simulink model "simRelativeNavSurfelGridMap"  (R2020b)
settings: Solver=FixedStepAuto  StartTime=0.0  StopTime=tEnd  FixedStep=dtSim  RelTol=1e-3
values from neighbouring files (symbols this model uses):
  flagUseTrueRelStates = 0    [testEnvironmentV2.m]    (also in testEnvironments.m = 1; testEnvironmentsV2.m; testEnvironmentsV3.m)
  fLArrayDim = size(fL1MeasArrayDir,1)    [SurfelGridMap.m]    (also in testEnvironmentV2.m = 256; testEnvironments.m = 256; testEnvironmentsV2.m = 256; testEnvironmentsV3.m = 256)
undefined symbols (not defined in the file or in its folder): angRate_IT_T, covMeasNoise, covProcessNoise, dtSim, fL1Pose_B, flagGravityAlignedNode, initCovState, initX, paramSGM, posi_TL_T, quat_TL, tEnd
libraries: IMUUnit x1, flashLiDARUnit x1
(part 2 of 2)

== matlab function simRelativeNavSurfelGridMap/RNerrorStateKalmanFilter ==
  settings: updateMethod=DISCRETE  sampleTime=dtSim
  data: accMeas input size=[3,1]; Xn output size=[10,1]; angRateMeas input size=[3,1]; deltaX_m input size=[7,1]; flagRegFinished input size=1; Pe output size=[9,9]; flagNewNode input boolean size=1; flagGravityAlignedNode input size=1; gravity_T input size=[3,1]; Xn_old_node output size=[10,1]; Pe_old_node output size=[9,9]; Xn_prop output size=[10,1]; angRate_IT_T parameter size=[3,1]; quat_TL parameter size=[4,1]; posi_TL_T parameter size=[3,1]; covMeasNoise parameter size=[6,6]; covProcessNoise parameter size=[9,9]; dtSim parameter size=1; initX parameter size=[10,1]; initCovState parameter size=[9,9]; acc_N output size=[3,1]; angRate_NB_B output size=[3,1]; posi_N1N2_N1_out output size=[3,1]; R_N1N2_out output size=[3,3]; R_N_fixed_out output size=[3,3]; R_LN_out output size=[3,3]; posi_LN_L_out output size=[3,1]; residual output size=[6,1]; flagStateUpdated output
function [Xn, Pe, Xn_old_node, Pe_old_node, Xn_prop, acc_N, angRate_NB_B,...
    posi_N1N2_N1_out, R_N1N2_out, R_N_fixed_out, R_LN_out, posi_LN_L_out,...
    residual, flagStateUpdated] = ...
    RNerrorStateKalmanFilter(accMeas, angRateMeas, deltaX_m,...
    flagRegFinished, flagNewNode, flagGravityAlignedNode, gravity_T,...                                 % inputs
    angRate_IT_T, quat_TL, posi_TL_T, covMeasNoise, covProcessNoise,...
    dtSim, initX, initCovState)...                                 % parameters

%% === initialization
persistent Xn_last Xe_last Pe_last Xn_fixed first_run first_scan posi_N1N2_N1 R_N1N2 R_N_fixed R_LN posi_LN_L;
% Xn_last; %nominal states of S/C from last iteration {10x1}
% Xe_last; %error states of the filter from last iteration {9x1}
% Pe_last; %error covariance matrix of the filter from last iteration {9x9}
% Xn_fixed; % fixed frame w.r.t. new node frame

if isempty(Xn_last), Xn_last = initX;end
if isempty(Xe_last), Xe_last = zeros(15,1);end
if isempty(Pe_last), Pe_last = initCovState;end
if isempty(Xn_fixed), Xn_fixed = initX;end
if isempty(first_run), first_run = 0;end
if isempty(first_scan), first_scan = 1;end

if isempty(posi_N1N2_N1), posi_N1N2_N1 = zeros(3,1);end
if isempty(R_N1N2), R_N1N2 = eye(3);end
if isempty(R_N_fixed), R_N_fixed = eye(3);end
if isempty(R_LN), R_LN = eye(3);end
if isempty(posi_LN_L), posi_LN_L = zeros(3,1);end

Xn = Xn_last;
Xe = zeros(9,1);
Pe = zeros(9);

Xn_old_node = Xn_last; % Xn before configuration of new node
Pe_old_node = zeros(9);
residual = zeros(6,1);
K = zeros(9,6);
posi_N1N2_N1_out = zeros(3,1);
R_N1N2_out = eye(3);
R_N_fixed_out = eye(3);
R_LN_out = eye(3);
posi_LN_L_out = zeros(3,1);
flagStateUpdated = 0;

R_TL = quat2rotmliub(quat_TL);


if(first_run > 0.5)
    Xn = Xn_last;
    Pe = zeros(9);
    
    Xn_old_node = Xn;
    Pe_old_node = Pe;
    Xn_prop = Xn;
    
    acc_N = zeros(3,1);
    angRate_NB_B = zeros(3,1);
    first_run = 0;
   return; 
end

q = Xn_last(7:10);
att_dcm_NB = [q(1)^2+q(4)^2-q(2)^2-q(3)^2 2*(q(1)*q(2)+q(3)*q(4))     2*(q(1)*q(3)-q(2)*q(4));
              2*(q(1)*q(2)-q(3)*q(4))     q(2)^2+q(4)^2-q(1)^2-q(3)^2 2*(q(2)*q(3)+q(1)*q(4));
              2*(q(1)*q(3)+q(2)*q(4))     2*(q(2)*q(3)-q(1)*q(4))     q(3)^2+q(4)^2-q(1)^2-q(2)^2];
% omega_IL_L = localFrameAtt_dcm_TL * angRate_IT_T;

angRate_IN_N = R_LN * R_TL * angRate_IT_T;

% IMU measurements acceleration and angular rate of body frame
% w.r.t inertial frame
accBias = 0;%Xn_last(11:13);
angRateBias = 0;%Xn_last(13:15);
acc_IB_B = accMeas - accBias;
angRate_IB_B = angRateMeas - angRateBias;


%% === INS propagation
Xn_prop = zeros(10,1);

%TODO!!!!!!
% after new node frame is configured,
% all terms in INS mechanization equations shall be transformed to the new
% node frame!!!-> using R_LN to relate L to node frame

prevPosi_NB_N = Xn_last(1:3);
prevVel_NB_N = Xn_last(4:6);
prevAtt_quat_NB = Xn_last(7:10);

% === translation
% calculate the effective gravitation
posi_LB_L = R_LN' * prevPosi_NB_N + posi_LN_L;
effGrav_T = gravity_T - cross(angRate_IT_T,cross(angRate_IT_T,posi_TL_T + R_TL'*posi_LB_L));

effGrav_N = R_LN * R_TL * effGrav_T;

acc_N = att_dcm_NB' * acc_IB_B + effGrav_N - 2 * cross(angRate_IN_N, prevVel_NB_N);

% Xn_pred(1:3) = prevPos_L + dt * prevVel_L + 0.5 * dt * dt * acc_L;
Xn_prop(1:3) = prevVel_NB_N * dtSim + prevPosi_NB_N;
Xn_prop(4:6) = acc_N * dtSim + prevVel_NB_N;

% === rotation
angRate_NB_B = angRate_IB_B - att_dcm_NB * angRate_IN_N;
Omega = [0                  angRate_NB_B(3)     -angRate_NB_B(2)	angRate_NB_B(1);
         -angRate_NB_B(3)	0                   angRate_NB_B(1)     angRate_NB_B(2);
         angRate_NB_B(2)	-angRate_NB_B(1)	0                   angRate_NB_B(3);
         -angRate_NB_B(1)	-angRate_NB_B(2)	-angRate_NB_B(3)	0];
qn_pred = 1/2 * dtSim * Omega *  prevAtt_quat_NB +  prevAtt_quat_NB;
qn_pred = qn_pred / norm(qn_pred);

Xn_prop(7:10) = qn_pred;

% TODO IMU biases
% Xn_prop(11:13) 
% Xn_prop(13:15) 


%% --- ESKF prediction
Xe_pred = zeros(9,1);
Pe_pred = zeros(9);
F = eye(9);
R_wdtt = eye(3);

% f [Xe_p, Pe_p]= errorPrediction(gyro_raw, acc_raw, att_dcm_LB,...
%     omega_IL_L, Pe_last, dt, covProcessNoise)

% covariance matrix of process noise in error state model
Ne = covProcessNoise;


% === position error
%e_position = e_position_old + dt * e_velocity_old;

% === velocity error
omega_IN_N_cross = [0               -angRate_IN_N(3)  angRate_IN_N(2);
                    angRate_IN_N(3)   0               -angRate_IN_N(1);
                    -angRate_IN_N(2)	angRate_IN_N(1)   0 ];

acc_raw = acc_IB_B;
acc_raw_cross = [0          -acc_raw(3)  acc_raw(2);
                 acc_raw(3)  0           -acc_raw(1);
                 -acc_raw(2) acc_raw(1)  0 ];
% e_velocity = -omega_LI_L_cross * omega_LI_L_cross * e_position_old * dt...
%     - 2 * omega_LI_L_cross * e_velocity_old * dt...
%     + att_dcm_LB' * acc_raw_cross * e_attitude_old * dt + e_velocity_old;

% === attitude error
wdt = dtSim * [angRate_IB_B(1) angRate_IB_B(2) angRate_IB_B(3)]';
theta_s = norm(wdt);
if(theta_s > 1e-10)
    vector_u = wdt / norm(wdt);
    u_cross = [0 -vector_u(3) vector_u(2);
                vector_u(3) 0 -vector_u(1);
                -vector_u(2) vector_u(1) 0];

    %according to "Quaternion kinematics for the error-state Kalman filter" of
    %Joan Sola, page 76
    R_wdtt = eye(3) - u_cross*sin(theta_s) + (vector_u * vector_u' - eye(3))*(1-cos(theta_s));
end

% e_attitude = R_wdtt * e_attitude_old;

% === error covariance matrix
%     F(1:3, 4:6) = dt * eye(3);
%     F(4:6, 7:9) = dt * att_dcm_LB' * acc_raw_cross;
%     F(7:9, 7:9) = R_wdtt;

% include Coriolis and centripetal terms
F(1:3, 4:6) = dtSim * eye(3);
F(4:6, 1:3) = -omega_IN_N_cross * omega_IN_N_cross * dtSim;
F(4:6, 4:6) = eye(3) - 2 * omega_IN_N_cross * dtSim;
F(4:6, 7:9) = dtSim * att_dcm_NB' * acc_raw_cross;
F(7:9, 7:9) = R_wdtt;

% TODO, F(10:15, 10:15)

%Xe_pred = F * Xe_last;
Pe_pred = F * Pe_last * F' + Ne;



%% --- ESKF update
Xe_up = zeros(9,1);
Pe_up = zeros(9);

Xn_cor =  zeros(10,1);
Xe_cor = zeros(9,1);
Pe_cor =  zeros(9);

Xn_r =  zeros(10,1);
Xe_r = zeros(9,1);
Pe_r =  zeros(9);

% === data preallocation
errorObserv = zeros(6,1);
% measurement covariance matrix that measures only position and quaternion
W = covMeasNoise;

% === main function
if(flagRegFinished < 0.5)
	%if point cloud preprocessing not finished
    %no observation for update arrives, only prediction
	Xn = Xn_prop;
    Xe = Xe_pred;
    Pe = Pe_pred;

else
    %if point cloud preprocessing finished
    if(first_scan > 0.5)
        Xn = Xn_prop;
        Xe = Xe_pred;
        Pe = Pe_pred;
        
        Xn_old_node = Xn;
        Pe_old_node = Pe;

        R_N_fixed = quat2rotmliub(Xn(7:10));      
        
        flagStateUpdated = 1;
        first_scan = 0;
        
        % === rest of system states, error states and error covariance
        % when new node frame is configured
        % question???
        % do we really need this in this part when(flagRegFinished <0.5)?
        if(flagNewNode >0.5)
            Xn_old_node = Xn;
            Pe_old_node = Pe;
            
            R_N1_cur = quat2rotmliub(Xn_old_node(7:10)); 
            eulAng_N1_cur = rotm2eulAngliub(R_N1_cur);

            % rotation matrix from current node frame to current fixed frame
            % differs only in roll and pitch            
            
            if(flagGravityAlignedNode < 0.5)
                %L-frame-z-axis aligned node
                eulAng_N1N2 = [0; 0; eulAng_N1_cur(3)];
                R_N1N2 = eulAng2rotmliub(eulAng_N1N2);
%                 eulAng_Nnew_cur = [eulAng_Nold_cur(1); eulAng_Nold_cur(2); 0];
%                 R_N_fixed = eulAng2rotmliub(eulAng_Nnew_cur);

            else
                %effective-gravity aligned node
%******************Baustelle
                % question??? reset of yaw angle, not completely follow gravity
                % vector but current body frame!!! would it be a problem???
                eulAng_N1N2_1 = [0; 0; eulAng_N1_cur(3)];
                R_N1N2_1 = eulAng2rotmliub(eulAng_N1N2_1);
                
                dir_N1 = [0 0 1]';
                dir_Grav = effGrav_N/norm(effGrav_N);
                rotAng = acos(dot(dir_N1, dir_Grav));
                rotaxis_temp = cross(dir_Grav, dir_N1);              
                rotaxis = rotaxis_temp / norm(rotaxis_temp);
                quat_N2_1Grav = [rotaxis * sin(rotAng/2); cos(rotAng/2)];
                R_N2_1Grav = quat2rotmliub(quat_N2_1Grav);
                R_N1N2 = R_N2_1Grav * R_N1N2_1;
                
%******************Baustelle
            end
            R_N_fixed = R_N1_cur * (R_N1N2)';
            eulAng_N2_cur = rotm2eulAngliub(R_N_fixed);

            % TODO!!!update translation and rotation from L frame to current node frame
            posi_N1N2_N1 = Xn_old_node(1:3);
            posi_LN_new = posi_LN_L + R_LN' * posi_N1N2_N1;
            posi_LN_L = posi_LN_new; % position from L to new N frame   
            R_LN_new = R_N1N2 * R_LN; % rotm from L to new N frame   
            R_LN = R_LN_new;

            % system states in new node frame
            % TODO!!!ATTENTION!!! here is the problem, velocity in body frame or node
            % frame!!!????? if in body frame, will be convenient
            Xn_r(1:3,1) = zeros(3,1);
            Xn_r(4:6,1) = R_N1N2 * Xn(4:6); % change velocity expressed in the new node frame
            Xn_r(7:10,1) = eulAng2quatliub(eulAng_N2_cur);

            Xn_fixed = Xn_r;
            Xe_r = zeros(9,1);

            % TODO according to Koch's paper
            U = zeros(9);
            U(4:6,4:6) = R_N1N2;
            Pe_r = U * Pe * U';

            % === output
            Xn = Xn_r;
            Xe = Xe_r;
            Pe = Pe_r;

        end
        

    else % real update
        He = zeros(6,9);
        He(1:3,1:3) = eye(3);%R_N_fixed;
        He(4:6,7:9) = 0.5 * eye(3);
                
        PHt = (He * Pe_pred)'; % Matlab is column-major, so (H*PX)' is more efficient than PX*H' [Tim 2004]
        S = He * PHt + W;
        
        % === compute virtual measurement
        deltaX_vir = zeros(7,1);
        deltaX_vir(1:3) = Xn_prop(1:3);
        deltaX_vir(4:7) = Xn_prop(7:10); % from node to current frame
        
        % === compute error observation with real and virtual measurements
        errorObserv(1:3) = deltaX_vir(1:3) - deltaX_m(1:3);
        
        qvir = deltaX_vir(4:7);
        qvirinv = [-qvir(1:3);qvir(4)];
        
        errorOb_q = quatMultiplication(qvirinv, deltaX_m(4:7));
        errorOb_deltaTheta = 2 * sign(errorOb_q(4)) * errorOb_q(1:3);
        
%         qu = residual_q(1:3);
%         qww = residual_q(4);
%         rn = qu / norm(qu);
%         thetaaa = 2*atan(norm(qu)/qww);
%         thetaa = rn * thetaaa;
        errorObserv(4:6) = errorOb_deltaTheta;
        
        % === compute residual
        residual = errorObserv - He * Xe_pred;
        
        % === compute Kalman gain
        K = PHt /(S);
        %K= PHt * inv(S);
        
        % === update error states
        Xe_up = K * residual;

        % === update error covariance matrix
        %P_u = P_p - K * H * P_p;%simplest form
        %P_u = P_p - K * S * K'; % symmetric form

        KH = K * He;
        I = eye(size(KH,1));
        Pe_up = (I-K*He) * Pe_pred * (I-K*He)' + K*W*K'; % symmetric and positive Joseph form

        % === correcte INS nominal states with updated error states
        Xn_cor(1:3) = Xn_prop(1:3) - Xe_up(1:3);
        Xn_cor(4:6) = Xn_prop(4:6) - Xe_up(4:6);

        theta_v = [Xe_up(7) Xe_up(8) Xe_up(9)]';
        theta_s = norm(theta_v);
        if(theta_s<1e-10)
            dq = [0 0 0 1]';
        else
            nv = theta_v/theta_s;
            dq = [nv * sin(0.5 * theta_s); cos(0.5 * theta_s)]; 
        end

        quat_up = quatMultiplication(Xn_prop(7:10),dq);
        quat_up = quat_up / norm(quat_up); % normalization
        Xn_cor(7:10) = quat_up;

        % TODO, Xn_cor(11:16)

        % === error state reset after update
        Xe_cor = zeros(9,1);
        G = eye(9);
    %         G(7:9,7:9) = eye(3) - 0.5 * [0 -Xe(9) Xe(8);
    %                                      Xe(9) 0 -Xe(7);
    %                                     -Xe(8) Xe(7) 0];
        Pe_cor = G * Pe_up * G';
        
        % === output
        Xn = Xn_cor;
        Xe = Xe_cor;
        Pe = Pe_cor;
        
        flagStateUpdated = 1;
        
        % === rest of system states, error states and error covariance
        % when new node frame is configured
        if(flagNewNode>0.5)
            Xn_old_node = Xn;
            Pe_old_node = Pe;
            R_N1_cur = quat2rotmliub(Xn_old_node(7:10)); 
            eulAng_N1_cur = rotm2eulAngliub(R_N1_cur);
            
            if(flagGravityAlignedNode < 0.5)
                %L-frame-z-axis aligned node
                
                % R_n1_n2 rotation matrix from old node to new node frame
                % differs only in yaw
                eulAng_N1N2 = [0; 0; eulAng_N1_cur(3)];
                R_N1N2 = eulAng2rotmliub(eulAng_N1N2);
                
%                 eulAng_Nnew_cur = [eulAng_Nold_cur(1); eulAng_Nold_cur(2); 0];
%                 R_N_fixed = eulAng2rotmliub(eulAng_Nnew_cur);

            else
                %effective-gravity aligned node
%******************Baustelle
            % question??? reset of yaw angle, not completely follow gravity
            % vector but current body frame!!! would it be a problem???
                eulAng_N1N2_1 = [0; 0; eulAng_N1_cur(3)];
                R_N1N2_1 = eulAng2rotmliub(eulAng_N1N2_1);
                
                dir_N1 = [0 0 1]';
                dir_Grav = effGrav_N/norm(effGrav_N);
                rotAng = acos(dot(dir_N1, dir_Grav));
                rotaxis_temp = cross(dir_Grav, dir_N1);              
                rotaxis = rotaxis_temp / norm(rotaxis_temp);
                quat_N2_1Grav = [rotaxis * sin(rotAng/2); cos(rotAng/2)];
                R_N2_1Grav = quat2rotmliub(quat_N2_1Grav);
                R_N1N2 = R_N2_1Grav * R_N1N2_1;
                
%******************Baustelle
            end
            
            % rotation matrix from current node frame to current fixed frame
            % differs only in roll and pitch
            R_N_fixed = R_N1_cur * (R_N1N2)';
            eulAng_N2_cur = rotm2eulAngliub(R_N_fixed);

            posi_N1N2_N1 = Xn_old_node(1:3);
            posi_LN_new = posi_LN_L + R_LN' * posi_N1N2_N1;
            posi_LN_L = posi_LN_new;
            R_LN_new = R_N1N2 * R_LN;
            R_LN = R_LN_new;
            
            % system states in new node frame
            % TODO!!!ATTENTION!!! here is the problem, velocity in body frame or node
            % frame!!!????? if in body frame, will be convenient
            Xn_r(1:3,1) = zeros(3,1);
            Xn_r(4:6,1) = R_N1N2 * Xn(4:6); % change velocity expressed in the new node frame
            Xn_r(7:10,1) = eulAng2quatliub(eulAng_N2_cur);

            Xn_fixed = Xn_r;
            Xe_r = zeros(9,1);
            
            % TODO according to Koch's paper
            U = zeros(9);
            U(4:6,4:6) = R_N1N2;
            Pe_r = U * Pe * U';
            
            % === output
            Xn = Xn_r;
            Xe = Xe_r;
            Pe = Pe_r;

        end
    end
end

%% --- output

Xn_last = Xn;
Xe_last = Xe;
Pe_last = Pe;

posi_N1N2_N1_out = posi_N1N2_N1;
R_N1N2_out = R_N1N2;
R_N_fixed_out = R_N_fixed;
R_LN_out = R_LN;
posi_LN_L_out = posi_LN_L;

end

== matlab function simRelativeNavSurfelGridMap/computeTrueRelState ==
  settings: updateMethod=DISCRETE  sampleTime=dtSim
  data: posi_LN_ref output size=[3,1]; R_LN_ref output size=[3,3]; truePose_LB input; trueAtt_eul_LB input; trueRelState output; flagNewNode input double size=1; gravity_input input; initX parameter size=[10,1]; flagGravityAlignedNode parameter size=1; quat_TL parameter; posi_TL_T parameter; angRate_IT_T parameter
function [posi_LN_ref, R_LN_ref, trueRelState] = computeTrueRelState(truePose_LB, trueAtt_eul_LB,...
                flagNewNode, gravity_input, initX, flagGravityAlignedNode,...
                quat_TL, posi_TL_T, angRate_IT_T)

persistent posi_LN R_LN;
if isempty(posi_LN), posi_LN = initX(1:3,1);end
if isempty(R_LN)
%     R_LN = quat2rotmliub(initX(7:10,1));
	R_LN = eye(3);
end

trueRelState = zeros(7,1);
posi_LN_ref = zeros(3,1);
R_LN_ref = eye(3);
R_TL = quat2rotmliub(quat_TL);

q_cur = eulAng2quatliub(trueAtt_eul_LB);

trueRelState(1:3,1) = R_LN * (truePose_LB - posi_LN);

q_LN = rotm2quatliub(R_LN);
q_inv = [-q_LN(1:3);q_LN(4)];
trueRelState(4:7,1) = quatMultiplication(q_inv,q_cur);

if(flagNewNode >0.5)
    posi_LN = truePose_LB;
    
    if(flagGravityAlignedNode<0.5)
        
        R_LN = eulAng2rotmliub([0 0 trueAtt_eul_LB(3)]);
    else
        %TODO what if flagGravityAlignedNode is used???
        R_LB = eulAng2rotmliub(trueAtt_eul_LB);
        R_N1B = R_LB * (R_LN');
        eulAng_N1B = rotm2eulAngliub(R_N1B);
        
        R_N1N2_1 = eulAng2rotmliub([0 0 eulAng_N1B(3)]);
        
        dir_N1 = [0 0 1]';
        effGrav_T = gravity_input - cross(angRate_IT_T,cross(angRate_IT_T,posi_TL_T + R_TL'*truePose_LB));
        effGrav_N1 = R_LN * R_TL * effGrav_T;
        dir_Grav = effGrav_N1/norm(effGrav_N1);
        rotAng = acos(dot(dir_N1, dir_Grav));
        rotaxis_temp = cross(dir_Grav, dir_N1);              
        rotaxis = rotaxis_temp / norm(rotaxis_temp);
        quat_N2_1Grav = [rotaxis * sin(rotAng/2); cos(rotAng/2)];
        R_N2_1Grav = quat2rotmliub(quat_N2_1Grav);
        R_N1N2 = R_N2_1Grav * R_N1N2_1;
        
        R_LN_new = R_N1N2 * R_LN;
        R_LN = R_LN_new;
    end

end

posi_LN_ref = posi_LN;
R_LN_ref = R_LN;
end
